simulink model "Subsystem"  (R2020b)
settings: Solver=FixedStepAuto  StartTime=0.0  StopTime=3.0  FixedStep=0.06  RelTol=1e-3
settings Model: Creator=nadee  LastModifiedBy=nadee
settings DataIOCC: SaveOutput=off  SaveTime=off

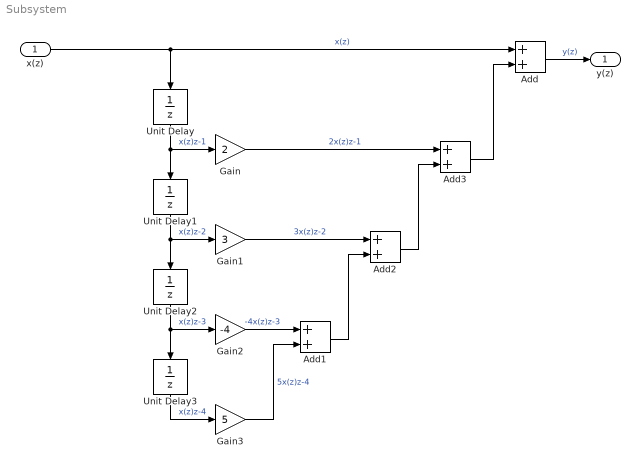
== system Subsystem ==
  x(z) : Inport  OutDataTypeStr=double  PortDimensions=1  SampleTime=[0.059999999999999998,0]
  Add{,1..3} (4 alike) : Sum
  Gain : Gain  Gain=2
  Gain1 : Gain  Gain=3
  Gain2 : Gain  Gain=-4
  Gain3 : Gain  Gain=5
  Unit Delay{,1..3} (4 alike) : UnitDelay  SampleTime=-1  HasFrameUpgradeWarning=on
  y(z) : Outport  OutDataTypeStr=double  PortDimensions=1  SampleTime=[0.059999999999999998,0]
  wires:
  Add1/1 -> Add2/2
  x(z)/1 -> Unit Delay/1, Add/1  "x(z)"
  Add/1 -> y(z)/1  "y(z)"
  Add2/1 -> Add3/2
  Unit Delay/1 -> Gain/1, Unit Delay1/1  "x(z)z-1"
  Unit Delay1/1 -> Gain1/1, Unit Delay2/1  "x(z)z-2"
  Add3/1 -> Add/2
  Unit Delay2/1 -> Gain2/1, Unit Delay3/1  "x(z)z-3"
  Gain3/1 -> Add1/2  "5x(z)z-4"
  Unit Delay3/1 -> Gain3/1  "x(z)z-4"
  Gain2/1 -> Add1/1  "-4x(z)z-3"
  Gain1/1 -> Add2/1  "3x(z)z-2"
  Gain/1 -> Add3/1  "2x(z)z-1"
